simulink model "parameters_estimation_ekf_dc"  (R2022b)
settings: Solver=ode1  StartTime=0.0  StopTime=10.0  FixedStep=0.001  RelTol=1e-3
settings Model: Creator=sokse  LastModifiedBy=sokse

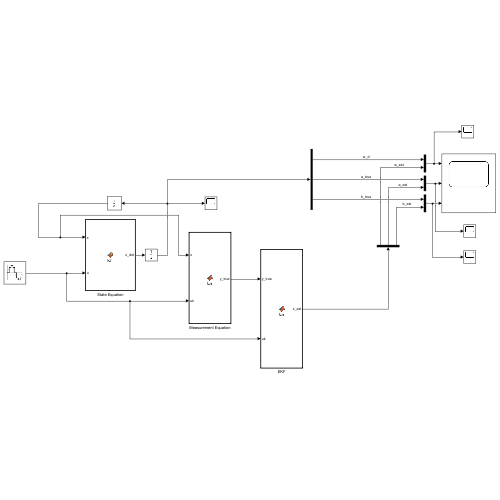
[thumbnail: Simulink's stored preview of the top-level diagram]
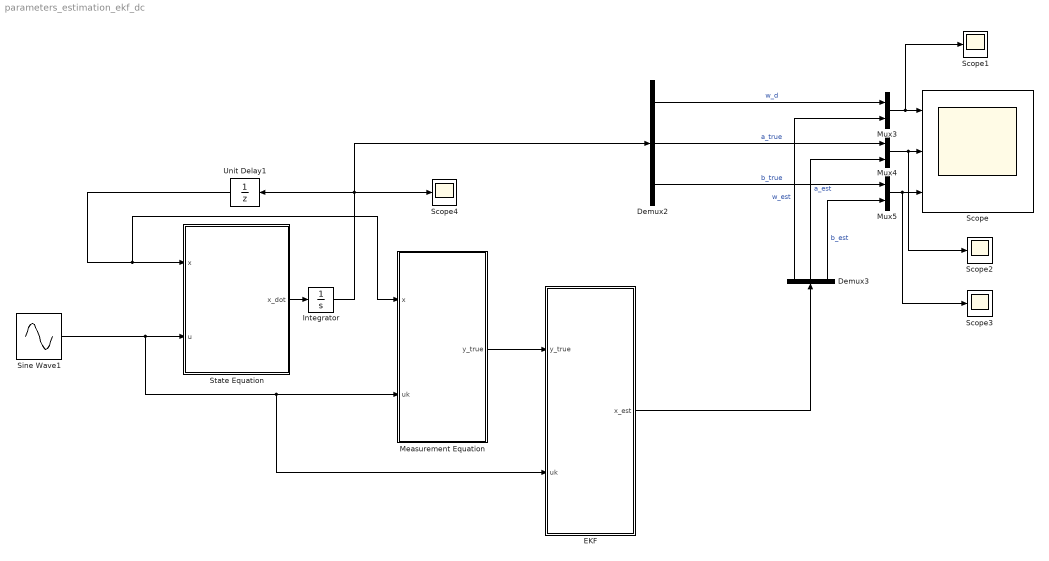
== system parameters_estimation_ekf_dc ==
  Demux2 : Demux  Outputs=3
  Demux3 : Demux  Outputs=3
  EKF : MATLAB Function  TreatAsAtomicUnit=on
  Integrator : Integrator  InitialCondition=[0;30.2;20.3]
  Measurement Equation : MATLAB Function  TreatAsAtomicUnit=on
  Mux3 : Mux  Inputs=2
  Mux4 : Mux  Inputs=2
  Mux5 : Mux  Inputs=2
  Scope : Scope  NumInputPorts=3
  Scope{1..4} (4 alike) : Scope
  Sine Wave1 : Sin  Amplitude=10  Frequency=2*pi*4  SampleTime=0.01  VectorParams1D=off
  State Equation : MATLAB Function  TreatAsAtomicUnit=on
  Unit Delay1 : UnitDelay  SampleTime=-1  HasFrameUpgradeWarning=on
  wires:
  State Equation/1(x_dot) -> Integrator/1
  Measurement Equation/1(y_true) -> EKF/1(y_true)
  Demux3/2 -> Mux4/2  "a_est"
  Demux2/3 -> Mux5/1  "b_true"
  Demux2/2 -> Mux4/1  "a_true"
  Demux3/1 -> Mux3/2  "w_est"
  Mux5/1 -> Scope3/1, Scope/3
  Demux3/3 -> Mux5/2  "b_est"
  Mux3/1 -> Scope1/1, Scope/1
  Mux4/1 -> Scope2/1, Scope/2
  Demux2/1 -> Mux3/1  "w_d"
  EKF/1(x_est) -> Demux3/1
  Sine Wave1/1 -> EKF/2(uk), Measurement Equation/2(uk), State Equation/2(u)
  Integrator/1 -> Scope4/1, Demux2/1, Unit Delay1/1
  Unit Delay1/1 -> Measurement Equation/1(x), State Equation/1(x)

== matlab function parameters_estimation_ekf_dc/State Equation ==
  settings: updateMethod=DISCRETE
  data: x input; u input; x_dot output
function x_dot = fcn(x,u)

x_dot = [0;0;0];

x_dot(1) = -x(2)*x(1)+x(3)*u +sqrt(0.01)*randn; % sqrt(0.02)*randn is model noise
x_dot(2) = 0;
x_dot(3) = 0;

== matlab function parameters_estimation_ekf_dc/EKF ==
  data: y_true input; uk input; x_est output
function x_est = fcn(y_true,uk)

Ts = 0.001; %Time step 

%Initialize initial value 
persistent x_est_p P Qd_est R_est Qc_est; 
if isempty(x_est_p)
    x_est_p = [0;0;0]; %Inital value of state x
    P       = 1e1*diag([1,10,5]); % Variance matrix 
    Qc_est  = 1e-1*diag([1,10,10]); % Process noise (small = believe in model)
    Qd_est  = Ts*Qc_est; % Process noise discretized to discrete time
    R_est   = 0.1; % Measurement noise (small = believe measurement) 
end 

C  = [1 0 0];
D  = 0; 
Ck = C; 
Dk = D; 

%Compute Kalman Gain and Update predicted Value 
Wk    = P*Ck'/(Ck*P*Ck'+R_est); 
y_est = Ck*x_est_p + Dk*uk; 
x     = x_est_p+Wk.*(y_true-y_est); 


%Compute prediction at next time step 
x_est = x+Ts*[-x(2)*x(1)+uk*x(3);
                       0;
                       0]; 

%Update error covariance matrices 
P = P-Wk*Ck*P; 

%Define Ak 
Ak = eye(3)+Ts*[-x(2) -x(1)  uk;
                  0     0    0;
                  0     0    0];   % Jacobian Matrix 

P = Ak*P*Ak'+Qd_est; 
x_est_p = x_est;

== matlab function parameters_estimation_ekf_dc/Measurement Equation ==
  settings: updateMethod=DISCRETE
  data: x input; uk input; y_true output
function y_true = fcn(x,uk)

C = [1 0 0];
D = 0;

y_true = C*x + D*uk + sqrt(0.02)*randn; % sqrt(0.02)*randn is measurement noise
